simulink model "Lat"  (R2022a)
settings: Solver=VariableStepAuto  StartTime=0.0  StopTime=300  RelTol=1e-3
values from neighbouring files (symbols this model uses):
  A_latr_full1 = [-0.177734438941 -0.0444373772428 -0.0121054087904 0 0 -51.1997940132 17.4487210829 4.99834967095 1 0 191.620649636 -70.8039136866 ... (25 elements, 5x5)]    [matlab.mat]
  B_latr_full = [Yda     Ydr ... (first row only)    [Lateral.m]    (also in matlab.mat = [0  0.0317; 4.76  5.35; 0.266  -0.923; 0  0; 0  0])
  C_latr_full = eye(5)    [Lateral.m]    (also in matlab.mat = [1 0 0 0 0 0 1 0 0 0 0 0 ... (25 elements, 5x5)])
  D_latr_full = zeros(5,2)    [Lateral.m]    (also in matlab.mat = [0  0; 0  0; 0  0; 0  0; 0  0])
  gravity = 32.174    [Lateral.m]    (also in Longituidinal.m; matlab.mat)
libraries: cstblocks x3, simulink_extras x2, slpidlib x1
settings Model: Creator=Mohamed Ismail  LastModifiedBy=Mohamed Ismail

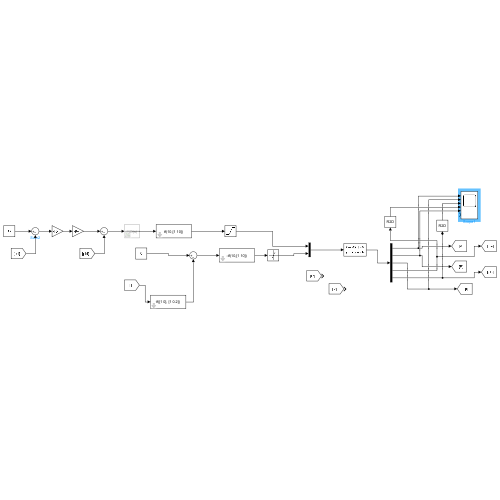
[thumbnail: Simulink's stored preview of the top-level diagram]
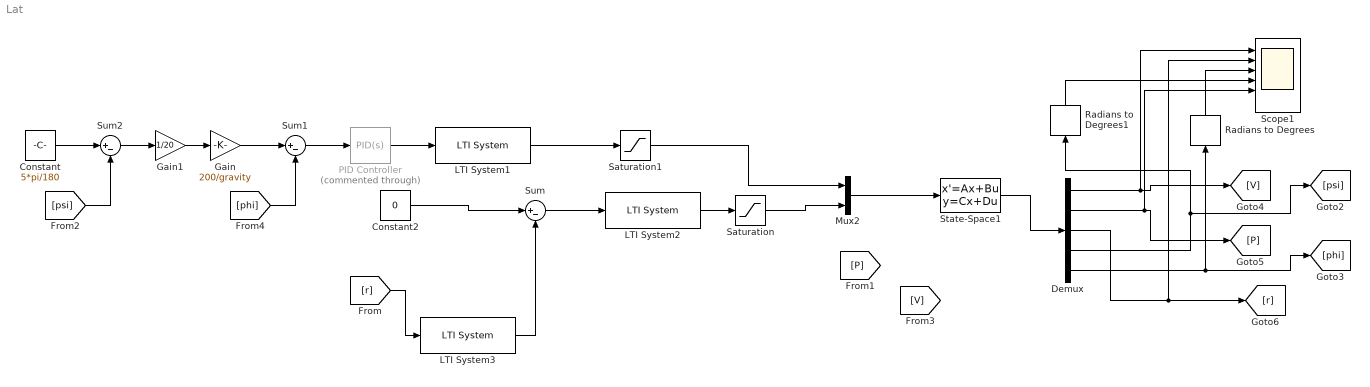
== system Lat ==
  Constant : Constant  Value=5*pi/180
  Constant2 : Constant  Value=0
  Demux : Demux  Outputs=5
  Gain : Gain  Gain=200/gravity
  Gain1 : Gain  Gain=1/20
  LTI System1 : cstblocks/LTI System  sys=tf(10,[1 10])  IC=[]
  LTI System2 : cstblocks/LTI System  sys=-tf(10,[1 10])  IC=[]
  LTI System3 : cstblocks/LTI System  sys=tf([1 0], [1 0.2])  IC=[]
  Mux2 : Mux  Inputs=2
  PID Controller : slpidlib/PID Controller  Commented=through  Controller=PID  Form=Parallel  TimeDomain=Continuous-time  UseExternalTs=off  SampleTime=-1  IntegratorMethod=Forward Euler  FilterMethod=Forward Euler  ControllerParametersSource=internal  P=0.363250528215049  I=0.0138253028436041  UseKiTs=off  D=2.12060034133301  N=745.569495243781  UseFilter=on  TunerSelectOption=Transfer Function Based (PID Tuner App)  InitialConditionSource=internal  InitialConditionForIntegrator=0  InitialConditionForFilter=0  DifferentiatorICPrevScaledInput=0  ExternalReset=none  TrackingMode=off  Kt=1  LimitOutput=off  SatLimitsSource=internal  UpperSaturationLimit=inf  LowerSaturationLimit=-inf  LinearizeAsGain=on  AntiWindupMode=none  Kb=1  POutMin=[]  POutMax=[]  IOutMin=[]  IOutMax=[]  DOutMin=[]  DOutMax=[]  NOutMin=[]  NOutMax=[]  SumOutMin=[]  SumOutMax=[]  SaturationOutMin=[]  SaturationOutMax=[]  PParamMin=[]  PParamMax=[]  IParamMin=[]  IParamMax=[]  DParamMin=[]  DParamMax=[]  NParamMin=[]  NParamMax=[]  KbParamMin=[]  KbParamMax=[]  KtParamMin=[]  KtParamMax=[]  KbOutMin=[]  KbOutMax=[]  KtOutMin=[]  KtOutMax=[]  IntegratorOutMin=[]  IntegratorOutMax=[]  FilterOutMin=[]  FilterOutMax=[]  SumI1OutMin=[]  SumI1OutMax=[]  SumI2OutMin=[]  SumI2OutMax=[]  SumI3OutMin=[]  SumI3OutMax=[]  SumI4OutMin=[]  SumI4OutMax=[]  SumDOutMin=[]  SumDOutMax=[]  DifferentiatorOutMin=[]  DifferentiatorOutMax=[]  FilterDiffOutCoefMin=[]  FilterDiffOutCoefMax=[]  ReciprocalOutMin=[]  ReciprocalOutMax=[]  SumDenOutMin=[]  SumDenOutMax=[]  SumNumOutMin=[]  SumNumOutMax=[]  DivideOutMin=[]  DivideOutMax=[]  UdiffTsProdOutMin=[]  UdiffTsProdOutMax=[]  NTsProdOutMin=[]  NTsProdOutMax=[]  UintegralTsProdOutMin=[]  UintegralTsProdOutMax=[]  UngainTsProdOutMin=[]  UngainTsProdOutMax=[]  IntegratorContinuousStateAttributes=''  IntegratorStateMustResolveToSignalObject=off  IntegratorRTWStateStorageClass=Auto  FilterContinuousStateAttributes=''  FilterStateMustResolveToSignalObject=off  FilterRTWStateStorageClass=Auto  ParallelPVariant=InternalParameters  IdealPVariant=Disabled  IVariant=InternalParameters  DVariant=InternalParameters  IntegratorVariant=Continuous  SatVariant=Disabled  AWVariant=Passthrough  PCopyVariant=Disabled  TRVariant=Disabled  FdbkBlocksVariant=Forward  IdealPFdbkVariant=Disabled  SatFdbkVariant=Disabled  DerivativeFilterVariant=ContFilter  NVariant=InternalParameters  NCopyVariant=Disabled  FilterICVariant=InternalICsFilter  IntegratorICVariant=InternalICs  ExternalResetVariant=Disabled  TRSumVariant=Passthrough  SumFdbkVariant=Disabled  SumVariant=Sum_PID  TsampFilterVariant=InternalTs  TsampNgainVariant=Passthrough  TsampIntegralVariant=Passthrough  ExternalSaturationOutDataTypeStr=Inherit: Same as second input  aMode=0
  Radians to Degrees : simulink_extras/Transformations/Radians to Degrees
  Radians to Degrees1 : simulink_extras/Transformations/Radians to Degrees
  Saturation : Saturate  UpperLimit=30*pi/180  LowerLimit=-30*pi/180
  Saturation1 : Saturate  UpperLimit=30*pi/180  LowerLimit=-30*pi/180  ZeroCross=off
  Scope1 : Scope  NumInputPorts=6
  State-Space1 : StateSpace  A=A_latr_full1  B=B_latr_full  C=C_latr_full  D=D_latr_full  InitialCondition=0  ParameterTunability=Unconstrained
  Sum : Sum  Inputs=|+-
  Sum1 : Sum  Inputs=|+-
  Sum2 : Sum  Inputs=|+-
  wires:
  State-Space1/1 -> Demux/1
  Saturation1/1 -> Mux2/1
  Mux2/1 -> State-Space1/1
  [phi] -> Sum1/2
  LTI System1/1 -> Saturation1/1
  Sum1/1 -> PID Controller/1
  Constant2/1 -> Sum/1
  [r] -> LTI System3/1
  LTI System2/1 -> Saturation/1
  Sum/1 -> LTI System2/1
  LTI System3/1 -> Sum/2
  Saturation/1 -> Mux2/2
  Radians to Degrees/1 -> Scope1/3
  Radians to Degrees1/1 -> Scope1/4
  PID Controller/1 -> LTI System1/1
  Demux/1 -> Scope1/1, [V]
  Demux/2 -> Scope1/5, [P]
  Demux/3 -> Scope1/2, [r]
  Demux/4 -> [psi], Radians to Degrees1/1
  Demux/5 -> Radians to Degrees/1, [phi]
  Gain/1 -> Sum1/1
  Gain1/1 -> Gain/1
  [psi] -> Sum2/2
  Constant/1 -> Sum2/1
  Sum2/1 -> Gain1/1
